simulink model "fitdf2filter_demo"  (Simulink 6.0)
settings: Solver=FixedStepDiscrete  StartTime=0.0  StopTime=n(end)  RelTol=1e-3
InitFcn:
  | ;
StartFcn:
  | ;
StopFcn:
  | ;
PreSaveFcn:
  | ;
CloseFcn:
  | ;
settings Model: Creator=tbryan  LastModifiedBy=tbryan  ExtModeAutoUpdateStatusClock=off
settings DataIOCC: SignalLoggingName=logsOut
settings DebuggingCC: CheckExecutionContextPreStartOutputMsg=on  CheckExecutionContextRuntimeOutputMsg=on  ParameterDowncastMsg=none  ParameterOverflowMsg=none  ParameterPrecisionLossMsg=none
settings SFSimCC: SFSimApplyToAllLibs=on  SFSimBuildMode=Incremental

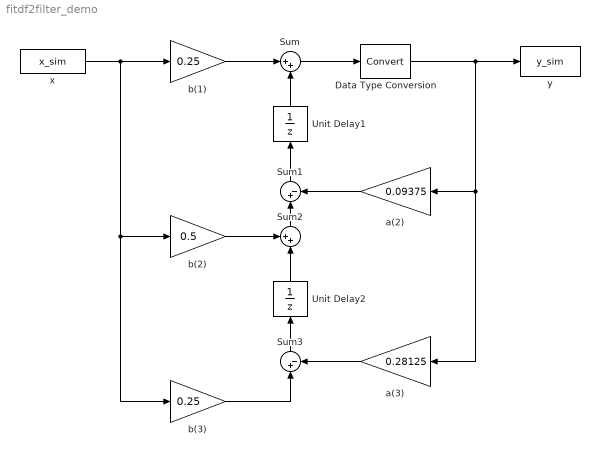
== system fitdf2filter_demo ==
  Data Type Conversion : DataTypeConversion  OutDataTypeMode=Specify via dialog  OutDataType=sfix(8)  OutScaling=2^-6  RndMeth=Nearest  SaturateOnIntegerOverflow=on  LockScale=on
  Sum : Sum  Inputs=|++  OutDataType=sfix(8)  OutScaling=2^-6  RndMeth=Nearest  SaturateOnIntegerOverflow=on
  Sum1 : Sum  Orientation=up  Inputs=|+-  OutDataType=sfix(8)  OutScaling=2^-6  RndMeth=Nearest  SaturateOnIntegerOverflow=on
  Sum2 : Sum  Orientation=up  Inputs=++|  RndMeth=Nearest  SaturateOnIntegerOverflow=on
  Sum3 : Sum  Orientation=up  Inputs=|+-  OutDataType=sfix(8)  OutScaling=2^-6  RndMeth=Nearest  SaturateOnIntegerOverflow=on
  Unit Delay1 : UnitDelay  Orientation=up
  Unit Delay2 : UnitDelay  Orientation=up
  a(2) : Gain  Orientation=left  Gain=0.09375  ParameterDataTypeMode=Specify via dialog  ParameterDataType=sfix(8)  ParameterScalingMode=Use specified scaling  ParameterScaling=2^-6  RndMeth=Nearest  SaturateOnIntegerOverflow=on
  a(3) : Gain  Orientation=left  Gain=0.28125  ParameterDataTypeMode=Specify via dialog  ParameterDataType=sfix(8)  ParameterScalingMode=Use specified scaling  ParameterScaling=2^-6  RndMeth=Nearest  SaturateOnIntegerOverflow=on
  b(1) : Gain  Gain=0.25  ParameterDataTypeMode=Specify via dialog  ParameterDataType=sfix(8)  ParameterScalingMode=Use specified scaling  ParameterScaling=2^-6  RndMeth=Nearest  SaturateOnIntegerOverflow=on
  b(2) : Gain  Gain=0.5  ParameterDataTypeMode=Specify via dialog  ParameterDataType=sfix(8)  ParameterScalingMode=Use specified scaling  ParameterScaling=2^-6  RndMeth=Nearest  SaturateOnIntegerOverflow=on
  b(3) : Gain  Gain=0.25  ParameterDataTypeMode=Specify via dialog  ParameterDataType=sfix(8)  ParameterScalingMode=Use specified scaling  ParameterScaling=2^-6  RndMeth=Nearest  SaturateOnIntegerOverflow=on
  x : FromWorkspace  VariableName=x_sim  SampleTime=0  Interpolate=off  OutputAfterFinalValue=Setting to zero
  y : ToWorkspace  VariableName=y_sim  SampleTime=-1  SaveFormat=Array
  wires:
  a(2)/1 -> Sum1/2
  b(2)/1 -> Sum2/1
  a(3)/1 -> Sum3/2
  Sum3/1 -> Unit Delay2/1
  Sum2/1 -> Sum1/1
  b(1)/1 -> Sum/1
  Unit Delay1/1 -> Sum/2
  x/1 -> b(2)/1, b(3)/1, b(1)/1
  Sum/1 -> Data Type Conversion/1
  b(3)/1 -> Sum3/1
  Data Type Conversion/1 -> y/1, a(3)/1, a(2)/1
  Unit Delay2/1 -> Sum2/2
  Sum1/1 -> Unit Delay1/1
